simulink model "gm_sampleModel1500_1_sub"  (R2023a)
settings: Solver=VariableStepAuto  StartTime=0.0  StopTime=10.0  RelTol=1e-3
libraries: hdlsllib x6, simulink x3
settings Model: Creator=user1  LastModifiedBy=user1
settings OptimizationCC: BlockReduction=off  ConditionallyExecuteInputs=off
settings DebuggingCC: InheritedTsInSrcMsg=none

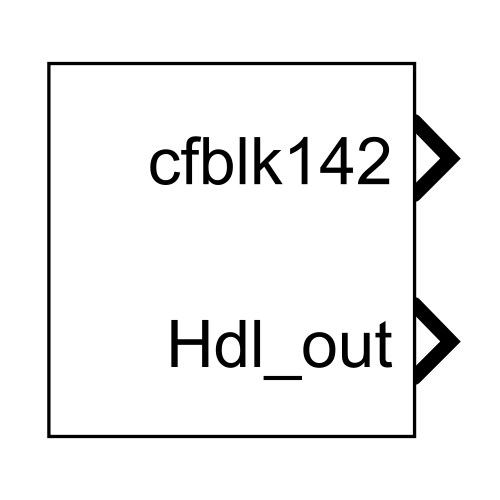
[thumbnail: Simulink's stored preview of the top-level diagram]
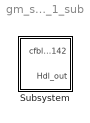
== system gm_sampleModel1500_1_sub ==
  Subsystem : Subsystem

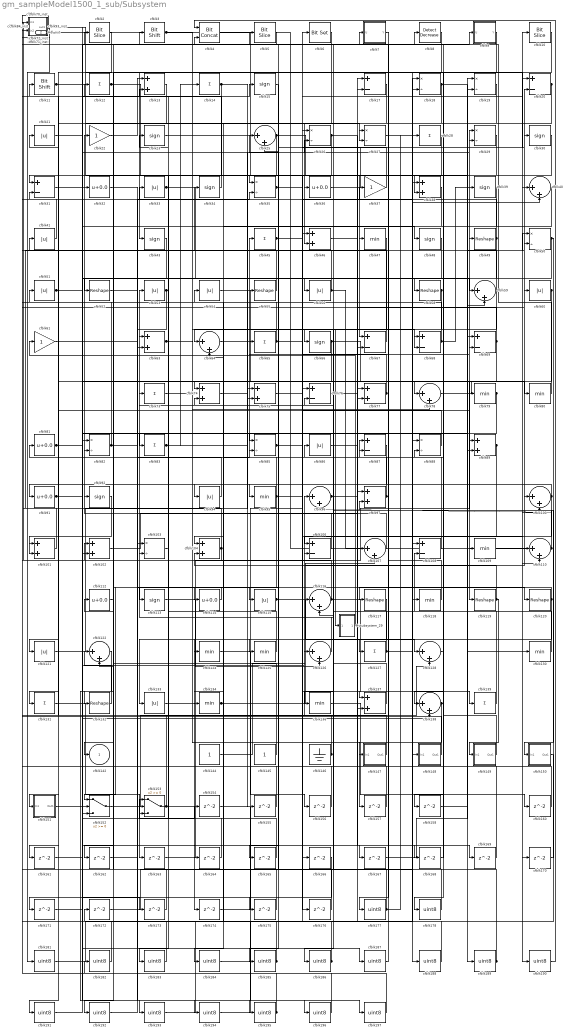
== system gm_sampleModel1500_1_sub/Subsystem ==
  Mysubsystem_29 : Subsystem
  cfblk10 : hdlsllib/Logic and Bit Operations/Bit Slice  lidx=7  ridx=0
  cfblk{25,40,59,64,78,96,100,107,110,116,122,126,128,138} (14 alike) : Sum  Inputs=|++  OutDataTypeStr=uint8
  cfblk{13,38,46,63,74..75,77,89,97,101..102,104,137} (13 alike) : Sum  OutDataTypeStr=uint8
  cfblk{18..19,26..27,29,35,50,82,85,88,103} (11 alike) : Product  Inputs=*/  OutDataTypeStr=uint8  RndMeth=Zero  SaturateOnIntegerOverflow=on
  cfblk105_inst : Subsystem
  cfblk{17,20,31,67..69,76,87,106,108} (10 alike) : Sum  Inputs=+-  OutDataTypeStr=uint8
  cfblk{47,79..80,95,109,118,124..125,130,134,136} (11 alike) : MinMax  OutDataTypeStr=uint8
  cfblk11 : hdlsllib/Logic and Bit Operations/Bit Shift  mode=Shift Left Logical  N=0
  cfblk{32,36,81,91,112,114} (6 alike) : Bias  Bias=0.0  SaturateOnIntegerOverflow=off
  cfblk{15,23,30,34,39,43,48,66,92,113} (10 alike) : Signum
  cfblk{21,33,41,51,53..54,56,60,86,94,115,121,133} (13 alike) : Abs  OutDataTypeStr=uint8  SaturateOnIntegerOverflow=off
  cfblk{49,52,55,58,117,119..120,132} (8 alike) : Reshape
  cfblk{12,14,28,45,65,73,83,127,131,139} (10 alike) : Sum  Inputs=+  OutDataTypeStr=uint8
  cfblk123_inst : Subsystem
  cfblk129_inst : Subsystem
  cfblk135_inst : Subsystem
  cfblk144 : Constant  OutDataTypeStr=uint8  SampleTime=-1
  cfblk145 : Constant  OutDataTypeStr=uint8  SampleTime=-1
  cfblk146 : Ground
  cfblk147 : Subsystem
  cfblk148 : Subsystem
  cfblk149 : Subsystem
  cfblk150 : Subsystem
  cfblk151 : Subsystem
  cfblk152 : Switch  OutDataTypeStr=uint8  SaturateOnIntegerOverflow=off  InputSameDT=off
  cfblk153 : Switch  OutDataTypeStr=uint8  SaturateOnIntegerOverflow=off  InputSameDT=off
  cfblk{154..158,160..176} (22 alike) : Delay  SampleTime=1
  cfblk16_inst : Subsystem
  cfblk{177..178,181..197} (19 alike) : DataTypeConversion  OutDataTypeStr=uint8  SaturateOnIntegerOverflow=off  RndMeth=Floor
  cfblk2 : hdlsllib/Logic and Bit Operations/Bit Slice  lidx=7  ridx=0
  cfblk22 : Gain  OutDataTypeStr=uint8
  cfblk24_inst : Subsystem
  cfblk3 : hdlsllib/Logic and Bit Operations/Bit Shift  mode=Shift Left Logical  N=0
  cfblk37 : Gain  OutDataTypeStr=uint8
  cfblk4 : hdlsllib/Logic and Bit Operations/Bit Concat  numInputs=2
  cfblk42_inst : Subsystem
  cfblk44_inst : Subsystem
  cfblk5 : hdlsllib/Logic and Bit Operations/Bit Slice  lidx=7  ridx=0
  cfblk57_inst : Subsystem
  cfblk6 : simulink/Logic and Bit Operations/Bit Set  iBit=0
      settings: LibrarySourceBlock=|
      | hdlsllib/Logic and Bit
      | Operations/Bit Set
  cfblk61 : Gain  OutDataTypeStr=uint8
  cfblk62_inst : Subsystem
  cfblk7 : Subsystem  mask(Detect Rise Nonnegative){vinit=double(0), InputProcessing=Elements as channels (sample based), OutDataTypeStr=uint8}
      mask prompts: vinit "Simulink:masks:InitialCondition_MP"; InputProcessing "Simulink:masks:InputProcessing_MP"; OutDataTypeStr "Simulink:masks:OutputDataType_MP"
      mask help: Simulink:masks:DetectRiseNonnegative_MD
      mask init:
      | InputProcessing = 'Elements as channels (sample based)';
      | OutDataTypeStr = 'uint8';
      | vinit = double(0);
      mask TypeOptions InputProcessing: Simulink:masks:ColumnsAsChannelsFrameBased | Simulink:masks:ElementsAsChannelsSampleBased
      mask TypeOptions OutDataTypeStr: Simulink:masks:uint8 | Simulink:masks:boolean
      mask Display: fprintf('U >= 0\n&  NOT\nU/z >= 0')
  cfblk70_inst : Subsystem
  cfblk71_inst : Subsystem
  cfblk72_inst : Subsystem
  cfblk8 : simulink/Logic and Bit Operations/Detect Decrease  vinit=0.0  OutDataTypeStr=uint8
      settings: LibrarySourceBlock=|
      | hdlsllib/Logic and Bit
      | Operations/Detect
      | Decrease
  cfblk84_inst : Subsystem
  cfblk9 : Subsystem  mask(Detect Rise Nonnegative){vinit=double(0), InputProcessing=Elements as channels (sample based), OutDataTypeStr=uint8}
      mask prompts: vinit "Simulink:masks:InitialCondition_MP"; InputProcessing "Simulink:masks:InputProcessing_MP"; OutDataTypeStr "Simulink:masks:OutputDataType_MP"
      mask help: Simulink:masks:DetectRiseNonnegative_MD
      mask init:
      | InputProcessing = 'Elements as channels (sample based)';
      | OutDataTypeStr = 'uint8';
      | vinit = double(0);
      mask TypeOptions InputProcessing: Simulink:masks:ColumnsAsChannelsFrameBased | Simulink:masks:ElementsAsChannelsSampleBased
      mask TypeOptions OutDataTypeStr: Simulink:masks:uint8 | Simulink:masks:boolean
      mask Display: fprintf('U >= 0\n&  NOT\nU/z >= 0')
  cfblk93_inst : Subsystem
  cfblk142 : Outport  OutDataTypeStr=uint8  SampleTime=1  VectorParamsAs1DForOutWhenUnconnected=off
  Hdl_out : Outport  Port=2  OutDataTypeStr=uint8  SampleTime=1
  wires:
  Mysubsystem_29/1(Out1) -> cfblk61/1
  cfblk10/1 -> cfblk43/1
  cfblk100/1 -> cfblk97/2, cfblk96/2, cfblk116/2, cfblk95/1
  cfblk101/1 -> cfblk20/2
  cfblk102/1 -> cfblk97/1
  cfblk103/1 -> cfblk33/1
  cfblk104/1 -> cfblk70_inst/1(in1), cfblk57_inst/2(in2)
  cfblk105_inst/1(out1) -> cfblk38/2
  cfblk106/1 -> cfblk22/1
  cfblk107/1 -> cfblk92/1
  cfblk108/1 -> cfblk45/1
  cfblk109/1 -> cfblk50/2
  cfblk11/1 -> cfblk46/2, cfblk36/1
  cfblk110/1 -> cfblk74/2, cfblk41/1, Hdl_out/1
  cfblk112/1 -> cfblk12/1
  cfblk113/1 -> cfblk126/2
  cfblk114/1 -> cfblk152/1
  cfblk115/1 -> cfblk128/1, cfblk107/2
  cfblk116/1 -> cfblk44_inst/1(in1), cfblk139/1
  cfblk117/1 -> cfblk133/1
  cfblk118/1 -> cfblk123_inst/1(in1)
  cfblk119/1 -> cfblk104/2, cfblk149/1(In1)
  cfblk12/1 -> cfblk27/2, cfblk166/1
  cfblk120/1 -> cfblk117/1, cfblk174/1
  cfblk121/1 -> cfblk75/1
  cfblk122/1 -> cfblk193/1
  cfblk123_inst/1(out1) -> cfblk84_inst/1(in1)
  cfblk124/1 -> cfblk156/1
  cfblk125/1 -> cfblk13/2
  cfblk126/1 -> cfblk53/1
  cfblk127/1 -> cfblk63/1, cfblk40/2
  cfblk128/1 -> cfblk8/1
  cfblk129_inst/1(out1) -> cfblk181/1
  cfblk13/1 -> cfblk162/1
  cfblk130/1 -> cfblk108/2
  cfblk131/1 -> cfblk163/1
  cfblk132/1 -> cfblk122/1
  cfblk133/1 -> cfblk29/1
  cfblk134/1 -> cfblk46/1, cfblk108/1
  cfblk135_inst/1(out1) -> cfblk40/1, cfblk32/1, cfblk148/1(In1)
  cfblk136/1 -> cfblk160/1
  cfblk137/1 -> cfblk73/1
  cfblk138/1 -> cfblk158/1, cfblk157/1
  cfblk139/1 -> cfblk3/1
  cfblk14/1 -> cfblk75/2, cfblk113/1
  cfblk144/1 -> cfblk110/1
  cfblk145/1 -> cfblk62_inst/1(in1)
  cfblk146/1 -> cfblk96/1, cfblk21/1
  cfblk147/1(Out1) -> cfblk112/1
  cfblk148/1(Out1) -> cfblk42_inst/2(in2)
  cfblk149/1(Out1) -> cfblk106/2
  cfblk15/1 -> cfblk85/1
  cfblk150/1(Out1) -> cfblk172/1
  cfblk151/1(Out1) -> cfblk126/1
  cfblk152/1 -> cfblk128/2
  cfblk153/1 -> cfblk72_inst/2(in2), cfblk26/1
  cfblk154/1 -> cfblk196/1
  cfblk155/1 -> cfblk42_inst/1(in1)
  cfblk156/1 -> cfblk71_inst/1(in1)
  cfblk157/1 -> cfblk116/1
  cfblk158/1 -> cfblk59/2
  cfblk16_inst/1(out1) -> cfblk70_inst/2(in2)
  cfblk160/1 -> cfblk105_inst/1(in1)
  cfblk161/1 -> cfblk153/1
  cfblk162/1 -> cfblk35/2
  cfblk163/1 -> cfblk77/1
  cfblk164/1 -> cfblk153/3
  cfblk165/1 -> cfblk103/2
  cfblk166/1 -> cfblk191/1
  cfblk167/1 -> cfblk19/2
  cfblk168/1 -> cfblk88/2
  cfblk169/1 -> cfblk82/2
  cfblk17/1 -> cfblk192/1
  cfblk170/1 -> cfblk100/1
  cfblk171/1 -> cfblk187/1
  cfblk172/1 -> cfblk18/2
  cfblk173/1 -> cfblk102/1
  cfblk174/1 -> cfblk20/1
  cfblk175/1 -> cfblk44_inst/2(in2)
  cfblk176/1 -> cfblk135_inst/2(in2)
  cfblk177/1 -> cfblk86/1, cfblk28/1
  cfblk178/1 -> cfblk7/1(U)
  cfblk18/1 -> cfblk52/1, cfblk27/1, cfblk175/1, cfblk125/1, cfblk130/1
  cfblk181/1 -> cfblk18/1
  cfblk182/1 -> cfblk129_inst/1(in1)
  cfblk183/1 -> cfblk129_inst/2(in2)
  cfblk184/1 -> cfblk6/1
  cfblk185/1 -> cfblk84_inst/2(in2), cfblk123_inst/2(in2)
  cfblk186/1 -> cfblk54/1, cfblk103/1
  cfblk187/1 -> cfblk87/1
  cfblk188/1 -> cfblk87/2
  cfblk189/1 -> cfblk25/2, cfblk82/1
  cfblk19/1 -> cfblk151/1(In1)
  cfblk190/1 -> cfblk4/1
  cfblk191/1 -> cfblk4/2
  cfblk192/1 -> cfblk154/1
  cfblk193/1 -> cfblk17/1
  cfblk194/1 -> cfblk17/2
  cfblk195/1 -> cfblk182/1, cfblk135_inst/1(in1)
  cfblk196/1 -> cfblk93_inst/1(in1)
  cfblk197/1 -> cfblk93_inst/2(in2)
  cfblk2/1 -> cfblk101/2
  cfblk20/1 -> cfblk64/1, cfblk122/2
  cfblk21/1 -> cfblk9/1(U)
  cfblk22/1 -> cfblk13/1
  cfblk23/1 -> cfblk76/1
  cfblk24_inst/1(out1) -> cfblk170/1
  cfblk25/1 -> cfblk67/1, cfblk121/1
  cfblk26/1 -> cfblk35/1, cfblk168/1
  cfblk27/1 -> cfblk118/1
  cfblk28/1 -> cfblk31/1
  cfblk29/1 -> cfblk83/1
  cfblk3/1 -> cfblk78/2, cfblk68/2
  cfblk30/1 -> cfblk171/1
  cfblk31/1 -> cfblk48/1
  cfblk32/1 -> cfblk194/1
  cfblk33/1 -> cfblk88/1, cfblk155/1
  cfblk34/1 -> cfblk62_inst/2(in2)
  cfblk35/1 -> cfblk68/1, cfblk137/1, cfblk167/1
  cfblk36/1 -> cfblk10/1
  cfblk37/1 -> cfblk72_inst/1(in1)
  cfblk38/1 -> cfblk184/1
  cfblk39/1 -> cfblk165/1
  cfblk4/1 -> cfblk189/1
  cfblk40/1 -> cfblk104/1
  cfblk41/1 -> cfblk31/2
  cfblk42_inst/1(out1) -> cfblk100/2
  cfblk43/1 -> cfblk102/2
  cfblk44_inst/1(out1) -> cfblk188/1
  cfblk45/1 -> cfblk37/1, cfblk47/1
  cfblk46/1 -> cfblk110/2
  cfblk47/1 -> cfblk94/1
  cfblk48/1 -> cfblk63/2
  cfblk49/1 -> cfblk58/1, cfblk16_inst/2(in2), cfblk138/1
  cfblk5/1 -> cfblk105_inst/2(in2)
  cfblk50/1 -> cfblk78/1, cfblk150/1(In1)
  cfblk51/1 -> cfblk56/1, cfblk29/2
  cfblk52/1 -> cfblk120/1
  cfblk53/1 -> cfblk23/1, cfblk153/2
  cfblk54/1 -> cfblk176/1
  cfblk55/1 -> cfblk34/1
  cfblk56/1 -> cfblk2/1, cfblk107/1
  cfblk57_inst/1(out1) -> cfblk138/2
  cfblk58/1 -> cfblk66/1, Mysubsystem_29/1(In1), cfblk136/1
  cfblk59/1 -> cfblk19/1, cfblk124/1
  cfblk6/1 -> cfblk185/1
  cfblk60/1 -> cfblk114/1, cfblk134/1
  cfblk61/1 -> cfblk197/1
  cfblk62_inst/1(out1) -> cfblk173/1
  cfblk63/1 -> cfblk77/2, cfblk183/1
  cfblk64/1 -> cfblk190/1
  cfblk65/1 -> cfblk71_inst/2(in2), cfblk69/2
  cfblk66/1 -> cfblk119/1, cfblk161/1
  cfblk67/1 -> cfblk24_inst/1(in1)
  cfblk68/1 -> cfblk5/1, cfblk39/1
  cfblk69/1 -> cfblk89/1, cfblk24_inst/2(in2), cfblk137/2
  cfblk7/1(Y) -> cfblk177/1
  cfblk70_inst/1(out1) -> cfblk152/2
  cfblk71_inst/1(out1) -> cfblk59/1
  cfblk72_inst/1(out1) -> cfblk169/1
  cfblk73/1 -> cfblk147/1(In1)
  cfblk74/1 -> cfblk49/1
  cfblk75/1 -> cfblk30/1
  cfblk76/1 -> cfblk38/1
  cfblk77/1 -> cfblk25/1, cfblk65/1
  cfblk78/1 -> cfblk80/1
  cfblk79/1 -> cfblk152/3, cfblk115/1
  cfblk8/1 -> cfblk132/1
  cfblk80/1 -> cfblk16_inst/1(in1)
  cfblk81/1 -> cfblk15/1, cfblk50/1
  cfblk82/1 -> cfblk57_inst/1(in1), cfblk11/1, cfblk85/2
  cfblk83/1 -> cfblk26/2, cfblk14/1
  cfblk84_inst/1(out1) -> cfblk89/2, cfblk74/1
  cfblk85/1 -> cfblk55/1, cfblk109/1
  cfblk86/1 -> cfblk69/1
  cfblk87/1 -> cfblk186/1
  cfblk88/1 -> cfblk51/1
  cfblk89/1 -> cfblk91/1, cfblk106/1
  cfblk9/1(Y) -> cfblk178/1
  cfblk91/1 -> cfblk164/1, cfblk131/1
  cfblk92/1 -> cfblk101/1
  cfblk93_inst/1(out1) -> cfblk195/1
  cfblk94/1 -> cfblk81/1
  cfblk95/1 -> cfblk64/2, cfblk142/1, cfblk79/1
  cfblk96/1 -> cfblk67/2, cfblk60/1
  cfblk97/1 -> cfblk76/2, cfblk127/1

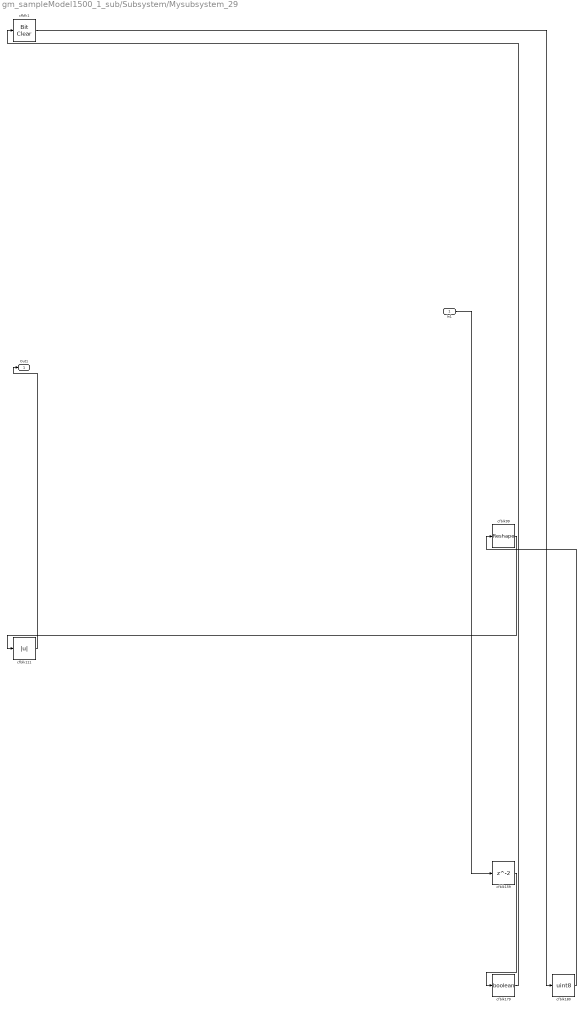
== system gm_sampleModel1500_1_sub/Subsystem/Mysubsystem_29 ==
  In1 : Inport  OutDataTypeStr=uint8  PortDimensions=1  SampleTime=1
  cfblk1 : simulink/Logic and Bit Operations/Bit Clear  iBit=0
      settings: LibrarySourceBlock=|
      | hdlsllib/Logic and Bit
      | Operations/Bit Clear
  cfblk111 : Abs  SaturateOnIntegerOverflow=off
  cfblk159 : Delay  SampleTime=1
  cfblk179 : DataTypeConversion  OutDataTypeStr=boolean  SaturateOnIntegerOverflow=off  RndMeth=Floor
  cfblk180 : DataTypeConversion  OutDataTypeStr=uint8  SaturateOnIntegerOverflow=off  RndMeth=Floor
  cfblk99 : Reshape
  Out1 : Outport  SampleTime=1
  wires:
  In1/1 -> cfblk159/1
  cfblk1/1 -> cfblk180/1
  cfblk111/1 -> Out1/1
  cfblk159/1 -> cfblk179/1
  cfblk179/1 -> cfblk1/1
  cfblk180/1 -> cfblk99/1
  cfblk99/1 -> cfblk111/1

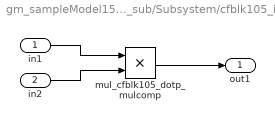
== system gm_sampleModel1500_1_sub/Subsystem/cfblk105_inst ==
  in1 : Inport  OutDataTypeStr=uint8  SampleTime=1
  in2 : Inport  Port=2  OutDataTypeStr=uint8  SampleTime=1
  mul_cfblk105_dotp_mulcomp : Product  Inputs=**  OutDataTypeStr=uint8  SampleTime=1
  out1 : Outport  OutDataTypeStr=uint8  SampleTime=1
  wires:
  in1/1 -> mul_cfblk105_dotp_mulcomp/1
  in2/1 -> mul_cfblk105_dotp_mulcomp/2
  mul_cfblk105_dotp_mulcomp/1 -> out1/1

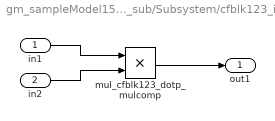
== system gm_sampleModel1500_1_sub/Subsystem/cfblk123_inst ==
  in1 : Inport  OutDataTypeStr=uint8  SampleTime=1
  in2 : Inport  Port=2  OutDataTypeStr=uint8  SampleTime=1
  mul_cfblk123_dotp_mulcomp : Product  Inputs=**  OutDataTypeStr=uint8  SampleTime=1
  out1 : Outport  OutDataTypeStr=uint8  SampleTime=1
  wires:
  in1/1 -> mul_cfblk123_dotp_mulcomp/1
  in2/1 -> mul_cfblk123_dotp_mulcomp/2
  mul_cfblk123_dotp_mulcomp/1 -> out1/1

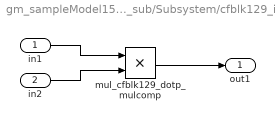
== system gm_sampleModel1500_1_sub/Subsystem/cfblk129_inst ==
  in1 : Inport  OutDataTypeStr=uint8  SampleTime=1
  in2 : Inport  Port=2  OutDataTypeStr=uint8  SampleTime=1
  mul_cfblk129_dotp_mulcomp : Product  Inputs=**  OutDataTypeStr=uint8  SampleTime=1
  out1 : Outport  OutDataTypeStr=uint8  SampleTime=1
  wires:
  in1/1 -> mul_cfblk129_dotp_mulcomp/1
  in2/1 -> mul_cfblk129_dotp_mulcomp/2
  mul_cfblk129_dotp_mulcomp/1 -> out1/1

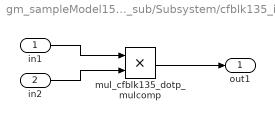
== system gm_sampleModel1500_1_sub/Subsystem/cfblk135_inst ==
  in1 : Inport  OutDataTypeStr=uint8  SampleTime=1
  in2 : Inport  Port=2  OutDataTypeStr=uint8  SampleTime=1
  mul_cfblk135_dotp_mulcomp : Product  Inputs=**  OutDataTypeStr=uint8  SampleTime=1
  out1 : Outport  OutDataTypeStr=uint8  SampleTime=1
  wires:
  in1/1 -> mul_cfblk135_dotp_mulcomp/1
  in2/1 -> mul_cfblk135_dotp_mulcomp/2
  mul_cfblk135_dotp_mulcomp/1 -> out1/1

== system gm_sampleModel1500_1_sub/Subsystem/cfblk147 ==
  In1 : Inport  OutDataTypeStr=uint8  PortDimensions=1  SampleTime=1
  Out1 : Outport  SampleTime=1
  wires:
  In1/1 -> Out1/1

== system gm_sampleModel1500_1_sub/Subsystem/cfblk148 ==
  In1 : Inport  OutDataTypeStr=uint8  PortDimensions=1  SampleTime=1
  Out1 : Outport  SampleTime=1
  wires:
  In1/1 -> Out1/1

== system gm_sampleModel1500_1_sub/Subsystem/cfblk149 ==
  In1 : Inport  OutDataTypeStr=uint8  PortDimensions=1  SampleTime=1
  Out1 : Outport  SampleTime=1
  wires:
  In1/1 -> Out1/1

== system gm_sampleModel1500_1_sub/Subsystem/cfblk150 ==
  In1 : Inport  OutDataTypeStr=uint8  PortDimensions=1  SampleTime=1
  Out1 : Outport  SampleTime=1
  wires:
  In1/1 -> Out1/1

== system gm_sampleModel1500_1_sub/Subsystem/cfblk151 ==
  In1 : Inport  OutDataTypeStr=uint8  PortDimensions=1  SampleTime=1
  Out1 : Outport  SampleTime=1
  wires:
  In1/1 -> Out1/1

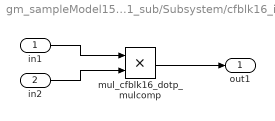
== system gm_sampleModel1500_1_sub/Subsystem/cfblk16_inst ==
  in1 : Inport  OutDataTypeStr=uint8  SampleTime=1
  in2 : Inport  Port=2  OutDataTypeStr=uint8  SampleTime=1
  mul_cfblk16_dotp_mulcomp : Product  Inputs=**  OutDataTypeStr=uint8  SampleTime=1
  out1 : Outport  OutDataTypeStr=uint8  SampleTime=1
  wires:
  in1/1 -> mul_cfblk16_dotp_mulcomp/1
  in2/1 -> mul_cfblk16_dotp_mulcomp/2
  mul_cfblk16_dotp_mulcomp/1 -> out1/1

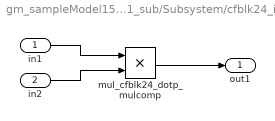
== system gm_sampleModel1500_1_sub/Subsystem/cfblk24_inst ==
  in1 : Inport  OutDataTypeStr=uint8  SampleTime=1
  in2 : Inport  Port=2  OutDataTypeStr=uint8  SampleTime=1
  mul_cfblk24_dotp_mulcomp : Product  Inputs=**  OutDataTypeStr=uint8  SampleTime=1
  out1 : Outport  OutDataTypeStr=uint8  SampleTime=1
  wires:
  in1/1 -> mul_cfblk24_dotp_mulcomp/1
  in2/1 -> mul_cfblk24_dotp_mulcomp/2
  mul_cfblk24_dotp_mulcomp/1 -> out1/1

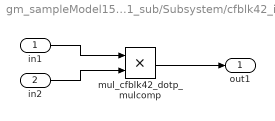
== system gm_sampleModel1500_1_sub/Subsystem/cfblk42_inst ==
  in1 : Inport  OutDataTypeStr=uint8  SampleTime=1
  in2 : Inport  Port=2  OutDataTypeStr=uint8  SampleTime=1
  mul_cfblk42_dotp_mulcomp : Product  Inputs=**  OutDataTypeStr=uint8  SampleTime=1
  out1 : Outport  OutDataTypeStr=uint8  SampleTime=1
  wires:
  in1/1 -> mul_cfblk42_dotp_mulcomp/1
  in2/1 -> mul_cfblk42_dotp_mulcomp/2
  mul_cfblk42_dotp_mulcomp/1 -> out1/1

== system gm_sampleModel1500_1_sub/Subsystem/cfblk44_inst ==
  in1 : Inport  OutDataTypeStr=uint8  SampleTime=1
  in2 : Inport  Port=2  OutDataTypeStr=uint8  SampleTime=1
  mul_cfblk44_dotp_mulcomp : Product  Inputs=**  OutDataTypeStr=uint8  SampleTime=1
  out1 : Outport  OutDataTypeStr=uint8  SampleTime=1
  wires:
  in1/1 -> mul_cfblk44_dotp_mulcomp/1
  in2/1 -> mul_cfblk44_dotp_mulcomp/2
  mul_cfblk44_dotp_mulcomp/1 -> out1/1

== system gm_sampleModel1500_1_sub/Subsystem/cfblk57_inst ==
  in1 : Inport  OutDataTypeStr=uint8  SampleTime=1
  in2 : Inport  Port=2  OutDataTypeStr=uint8  SampleTime=1
  mul_cfblk57_dotp_mulcomp : Product  Inputs=**  OutDataTypeStr=uint8  SampleTime=1
  out1 : Outport  OutDataTypeStr=uint8  SampleTime=1
  wires:
  in1/1 -> mul_cfblk57_dotp_mulcomp/1
  in2/1 -> mul_cfblk57_dotp_mulcomp/2
  mul_cfblk57_dotp_mulcomp/1 -> out1/1

== system gm_sampleModel1500_1_sub/Subsystem/cfblk62_inst ==
  in1 : Inport  OutDataTypeStr=uint8  SampleTime=1
  in2 : Inport  Port=2  OutDataTypeStr=uint8  SampleTime=1
  mul_cfblk62_dotp_mulcomp : Product  Inputs=**  OutDataTypeStr=uint8  SampleTime=1
  out1 : Outport  OutDataTypeStr=uint8  SampleTime=1
  wires:
  in1/1 -> mul_cfblk62_dotp_mulcomp/1
  in2/1 -> mul_cfblk62_dotp_mulcomp/2
  mul_cfblk62_dotp_mulcomp/1 -> out1/1

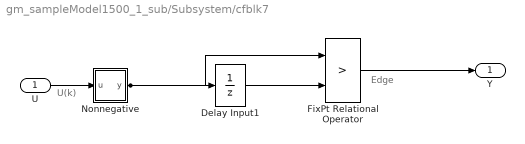
== system gm_sampleModel1500_1_sub/Subsystem/cfblk7 ==
  note: U(k)
  note: Edge
  U : Inport  OutDataTypeStr=uint8  SampleTime=1
  Delay Input1 : UnitDelay  Description=Store in Global RAM  DisableCoverage=on  InitialCondition=vinit  SampleTime=-1  HasFrameUpgradeWarning=on
  FixPt Relational Operator : RelationalOperator  Operator=>  OutDataTypeStr=fixdt(0, 8)  ZeroCross=off  InputSameDT=off
  Nonnegative : Subsystem  mask(Compare To Zero){relop=>=, OutDataTypeStr=boolean, ZeroCross=off}
      mask prompts: relop "Simulink:masks:Operator_MP"; OutDataTypeStr "Simulink:masks:OutputDataType_MP"; ZeroCross "Simulink:masks:EnableZerocrossingDetection_MP"
      mask help: Simulink:masks:CompareToZero_MD
      mask init:
      | OutDataTypeStr = 'boolean';
      | ZeroCross = 'off';
      | blkName = 'sampleModel1500_1_sub/Subsystem/cfblk7/Nonnegative';
      | relop = '>=';
      | setValue = 'boolean';
      mask TypeOptions relop: == | ~= | < | <= | >= | >
      mask TypeOptions OutDataTypeStr: Simulink:masks:uint8 | Simulink:masks:boolean
      mask Callback ZeroCross: sl('zeroCrossEnable', gcbh);
      mask Display: disp([relop,' 0'])
  Y : Outport  SampleTime=1
  wires:
  U/1 -> Nonnegative/1(u)
  Delay Input1/1 -> FixPt Relational Operator/2
  FixPt Relational Operator/1 -> Y/1
  Nonnegative/1(y) -> FixPt Relational Operator/1, Delay Input1/1

== system gm_sampleModel1500_1_sub/Subsystem/cfblk70_inst ==
  in1 : Inport  OutDataTypeStr=uint8  SampleTime=1
  in2 : Inport  Port=2  OutDataTypeStr=uint8  SampleTime=1
  mul_cfblk70_dotp_mulcomp : Product  Inputs=**  OutDataTypeStr=uint8  SampleTime=1
  out1 : Outport  OutDataTypeStr=uint8  SampleTime=1
  wires:
  in1/1 -> mul_cfblk70_dotp_mulcomp/1
  in2/1 -> mul_cfblk70_dotp_mulcomp/2
  mul_cfblk70_dotp_mulcomp/1 -> out1/1

== system gm_sampleModel1500_1_sub/Subsystem/cfblk71_inst ==
  in1 : Inport  OutDataTypeStr=uint8  SampleTime=1
  in2 : Inport  Port=2  OutDataTypeStr=uint8  SampleTime=1
  mul_cfblk71_dotp_mulcomp : Product  Inputs=**  OutDataTypeStr=uint8  SampleTime=1
  out1 : Outport  OutDataTypeStr=uint8  SampleTime=1
  wires:
  in1/1 -> mul_cfblk71_dotp_mulcomp/1
  in2/1 -> mul_cfblk71_dotp_mulcomp/2
  mul_cfblk71_dotp_mulcomp/1 -> out1/1

== system gm_sampleModel1500_1_sub/Subsystem/cfblk72_inst ==
  in1 : Inport  OutDataTypeStr=uint8  SampleTime=1
  in2 : Inport  Port=2  OutDataTypeStr=uint8  SampleTime=1
  mul_cfblk72_dotp_mulcomp : Product  Inputs=**  OutDataTypeStr=uint8  SampleTime=1
  out1 : Outport  OutDataTypeStr=uint8  SampleTime=1
  wires:
  in1/1 -> mul_cfblk72_dotp_mulcomp/1
  in2/1 -> mul_cfblk72_dotp_mulcomp/2
  mul_cfblk72_dotp_mulcomp/1 -> out1/1

== system gm_sampleModel1500_1_sub/Subsystem/cfblk84_inst ==
  in1 : Inport  OutDataTypeStr=uint8  SampleTime=1
  in2 : Inport  Port=2  OutDataTypeStr=uint8  SampleTime=1
  mul_cfblk84_dotp_mulcomp : Product  Inputs=**  OutDataTypeStr=uint8  SampleTime=1
  out1 : Outport  OutDataTypeStr=uint8  SampleTime=1
  wires:
  in1/1 -> mul_cfblk84_dotp_mulcomp/1
  in2/1 -> mul_cfblk84_dotp_mulcomp/2
  mul_cfblk84_dotp_mulcomp/1 -> out1/1

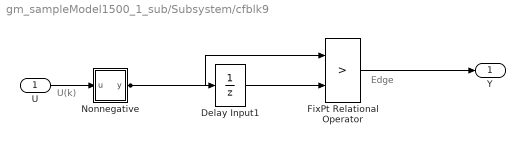
== system gm_sampleModel1500_1_sub/Subsystem/cfblk9 ==
  note: U(k)
  note: Edge
  U : Inport  OutDataTypeStr=uint8  SampleTime=1
  Delay Input1 : UnitDelay  Description=Store in Global RAM  DisableCoverage=on  InitialCondition=vinit  SampleTime=-1  HasFrameUpgradeWarning=on
  FixPt Relational Operator : RelationalOperator  Operator=>  OutDataTypeStr=fixdt(0, 8)  ZeroCross=off  InputSameDT=off
  Nonnegative : Subsystem  mask(Compare To Zero){relop=>=, OutDataTypeStr=boolean, ZeroCross=off}
      mask prompts: relop "Simulink:masks:Operator_MP"; OutDataTypeStr "Simulink:masks:OutputDataType_MP"; ZeroCross "Simulink:masks:EnableZerocrossingDetection_MP"
      mask help: Simulink:masks:CompareToZero_MD
      mask init:
      | OutDataTypeStr = 'boolean';
      | ZeroCross = 'off';
      | blkName = 'sampleModel1500_1_sub/Subsystem/cfblk9/Nonnegative';
      | relop = '>=';
      | setValue = 'boolean';
      mask TypeOptions relop: == | ~= | < | <= | >= | >
      mask TypeOptions OutDataTypeStr: Simulink:masks:uint8 | Simulink:masks:boolean
      mask Callback ZeroCross: sl('zeroCrossEnable', gcbh);
      mask Display: disp([relop,' 0'])
  Y : Outport  SampleTime=1
  wires:
  U/1 -> Nonnegative/1(u)
  Delay Input1/1 -> FixPt Relational Operator/2
  FixPt Relational Operator/1 -> Y/1
  Nonnegative/1(y) -> FixPt Relational Operator/1, Delay Input1/1

== system gm_sampleModel1500_1_sub/Subsystem/cfblk93_inst ==
  in1 : Inport  OutDataTypeStr=uint8  SampleTime=1
  in2 : Inport  Port=2  OutDataTypeStr=uint8  SampleTime=1
  mul_cfblk93_dotp_mulcomp : Product  Inputs=**  OutDataTypeStr=uint8  SampleTime=1
  out1 : Outport  OutDataTypeStr=uint8  SampleTime=1
  wires:
  in1/1 -> mul_cfblk93_dotp_mulcomp/1
  in2/1 -> mul_cfblk93_dotp_mulcomp/2
  mul_cfblk93_dotp_mulcomp/1 -> out1/1

== system gm_sampleModel1500_1_sub/Subsystem/cfblk7/Nonnegative ==
  u : Inport  OutDataTypeStr=uint8  SampleTime=1
  Compare : RelationalOperator  OutDataTypeStr=boolean  ZeroCross=off
  Constant : Constant  DisableCoverage=on  Value=0  OutDataTypeStr=Inherit: Inherit via back propagation  SampleTime=-1  PreserveConstantTs=on
  y : Outport  SampleTime=1
  wires:
  u/1 -> Compare/1
  Compare/1 -> y/1
  Constant/1 -> Compare/2

== system gm_sampleModel1500_1_sub/Subsystem/cfblk9/Nonnegative ==
  u : Inport  OutDataTypeStr=uint8  SampleTime=1
  Compare : RelationalOperator  OutDataTypeStr=boolean  ZeroCross=off
  Constant : Constant  DisableCoverage=on  Value=0  OutDataTypeStr=Inherit: Inherit via back propagation  SampleTime=-1  PreserveConstantTs=on
  y : Outport  SampleTime=1
  wires:
  u/1 -> Compare/1
  Compare/1 -> y/1
  Constant/1 -> Compare/2
